simulink model "WindTurbine_PI_Final_Model"  (R2025a)
settings: Solver=VariableStepAuto  StartTime=0.0  StopTime=20  RelTol=1e-3
settings Model: Creator=hero  LastModifiedBy=hero

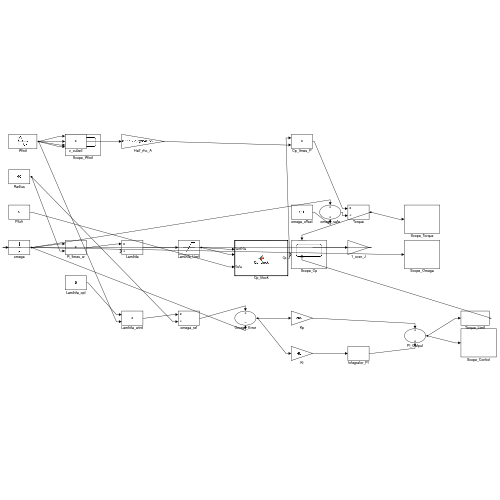
[thumbnail: Simulink's stored preview of the top-level diagram]
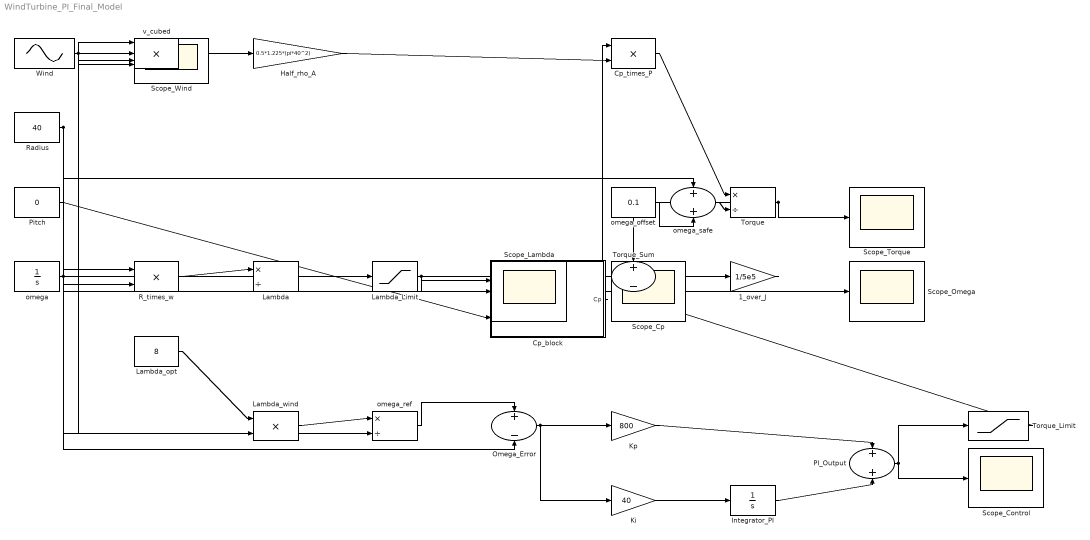
== system WindTurbine_PI_Final_Model ==
  1_over_J : Gain  Gain=1/5e5
  Cp_block : MATLAB Function  TreatAsAtomicUnit=on
  Cp_times_P : Product
  Half_rho_A : Gain  Gain=0.5*1.225*(pi*40^2)
  Integrator_PI : Integrator
  Ki : Gain  Gain=40
  Kp : Gain  Gain=800
  Lambda : Product  Inputs=*/
  Lambda_Limit : Saturate  UpperLimit=10  LowerLimit=2
  Lambda_opt : Constant  Value=8
  Lambda_wind : Product
  Omega_Error : Sum  Inputs=+-
  PI_Output : Sum
  Pitch : Constant  Value=0
  R_times_w : Product
  Radius : Constant  Value=40
  Scope_Control : Scope
  Scope_Cp : Scope
  Scope_Lambda : Scope
  Scope_Omega : Scope
  Scope_Torque : Scope
  Scope_Wind : Scope
  Torque : Product  Inputs=*/
  Torque_Limit : Saturate  UpperLimit=8e5  LowerLimit=0
  Torque_Sum : Sum  Inputs=+-
  Wind : Sin  Amplitude=2  Bias=10  Frequency=0.3  SampleTime=0
  omega : Integrator  InitialCondition=1
  omega_offset : Constant  Value=0.1
  omega_ref : Product  Inputs=*/
  omega_safe : Sum
  v_cubed : Product  Inputs=3
  wires:
  Wind/1 -> Scope_Wind/1, v_cubed/1, v_cubed/2, v_cubed/3, Lambda_wind/2
  omega/1 -> R_times_w/1, omega_safe/1, Scope_Omega/1, Omega_Error/2
  Radius/1 -> R_times_w/2, omega_ref/2
  R_times_w/1 -> Lambda/1
  Lambda/1 -> Lambda_Limit/1
  Lambda_Limit/1 -> Scope_Lambda/1, Cp_block/1(lambda)
  Pitch/1 -> Cp_block/2(beta)
  v_cubed/1 -> Half_rho_A/1
  Half_rho_A/1 -> Cp_times_P/2
  Cp_block/1(Cp) -> Cp_times_P/1
  omega_offset/1 -> omega_safe/2
  Cp_times_P/1 -> Torque/1
  omega_safe/1 -> Torque/2
  Torque/1 -> Scope_Torque/1, Torque_Sum/1
  Torque_Sum/1 -> 1_over_J/1
  1_over_J/1 -> omega/1
  Lambda_opt/1 -> Lambda_wind/1
  Lambda_wind/1 -> omega_ref/1
  omega_ref/1 -> Omega_Error/1
  Omega_Error/1 -> Kp/1, Ki/1
  Ki/1 -> Integrator_PI/1
  Kp/1 -> PI_Output/1
  Integrator_PI/1 -> PI_Output/2
  PI_Output/1 -> Scope_Control/1, Torque_Limit/1
  Torque_Limit/1 -> Torque_Sum/2

== matlab function WindTurbine_PI_Final_Model/Cp_block ==
  data: lambda input; Cp output; beta input
function Cp = Cp_block(lambda,beta)
lambda_i = 1/((1/(lambda+0.08*beta))-(0.035/(beta^3+1)));
Cp = 0.22*((116/lambda_i)-0.4*beta-5)*exp(-12.5/lambda_i);
Cp = max(0, Cp);
end
